simulink model "attempt_at_model_final"  (R2024a)
settings: Solver=FixedStepDiscrete  StartTime=0.0  StopTime=inf  FixedStep=0.01  RelTol=1e-3
model workspace (MAT data in the model file):
  SL_ROS_VariableLengthArrays_MaxSizes.CommonInfo.ArrayTruncateAction = 'EmitWarning'
  SL_ROS_VariableLengthArrays_MaxSizes.MsgTypeMap = containers.Map
  SL_ROS_VariableLengthArrays_MaxSizes.MsgTypeMap.serialization.keys = {'sensor_msgs/CompressedImage'}
  SL_ROS_VariableLengthArrays_MaxSizes.MsgTypeMap.serialization.values{1}(1).PropertyName = 'data'
  SL_ROS_VariableLengthArrays_MaxSizes.MsgTypeMap.serialization.values{1}(1).DataType = 'uint8'
  SL_ROS_VariableLengthArrays_MaxSizes.MsgTypeMap.serialization.values{1}(1).MaxLength = 87917
  SL_ROS_VariableLengthArrays_MaxSizes.MsgTypeMap.serialization.values{1}(2).PropertyName = 'format'
  SL_ROS_VariableLengthArrays_MaxSizes.MsgTypeMap.serialization.values{1}(2).DataType = 'uint8'
  SL_ROS_VariableLengthArrays_MaxSizes.MsgTypeMap.serialization.values{1}(2).MaxLength = 128
  SL_ROS_VariableLengthArrays_MaxSizes.MsgTypeMap.serialization.uniformity = 0
  SL_ROS_VariableLengthArrays_MaxSizes.MsgTypeMap.serialization.keyType = 'char'
  SL_ROS_VariableLengthArrays_MaxSizes.MsgTypeMap.serialization.valueType = 'any'
undefined symbols (not defined in the file): angular, linear
libraries: ros2lib x13, simulink x3, instrumentlib x1, etargetslib x1, vrlib x1, dspnetwork x1
settings Model: Creator=RedBlueBerry177  LastModifiedBy=ethan
settings OptimizationCC: EnhancedBackFolding=on  PassReuseOutputArgsAs=Individual arguments  ZeroExternalMemoryAtStartup=off  ZeroInternalMemoryAtStartup=off  MaxStackSize=64  OptimizeBlockOrder=speed  DifferentSizesBufferReuse=on  OptimizationCustomize=off  EfficientTunableParamExpr=on
settings DebuggingCC: ParameterTunabilityLossMsg=error
settings SFSimCC: MATLABDynamicMemAlloc=off  SimTargetLang=C++
settings RTWCC: Description=Embedded Coder  SystemTargetFile=ert.tlc  HardwareBoard=Robot Operating System 2 (ROS 2)  TLCOptions="-aInlineSetEventsForThisBaseRateFcn=TLC_FALSE -aSuppressMultiTaskScheduler=TLC_FALSE  -aRateBasedStepFcn=0"  TemplateMakefile=ert_default_tmf  Toolchain=Colcon Tools  TargetLang=C++  GPUComputeCapability=3.5
settings CodeAppCC: ForceParamTrailComments=on  IgnoreCustomStorageClasses=off  OperatorAnnotations=on  SimulinkDataObjDesc=on  SFDataObjDesc=on  InsertBlockDesc=on
settings ERTTargetCC: CodeInterfacePackaging=C++ class  RootIOFormat=Structure reference

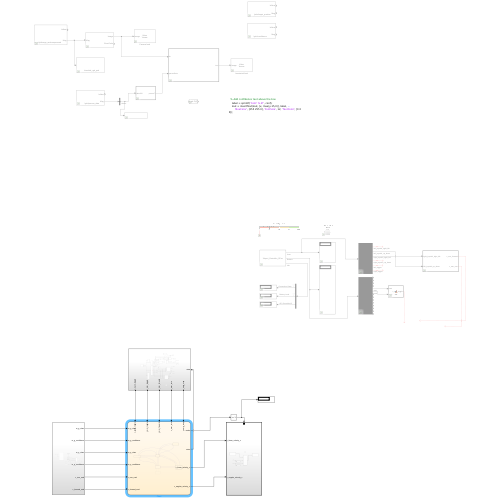
[thumbnail: Simulink's stored preview of the top-level diagram]
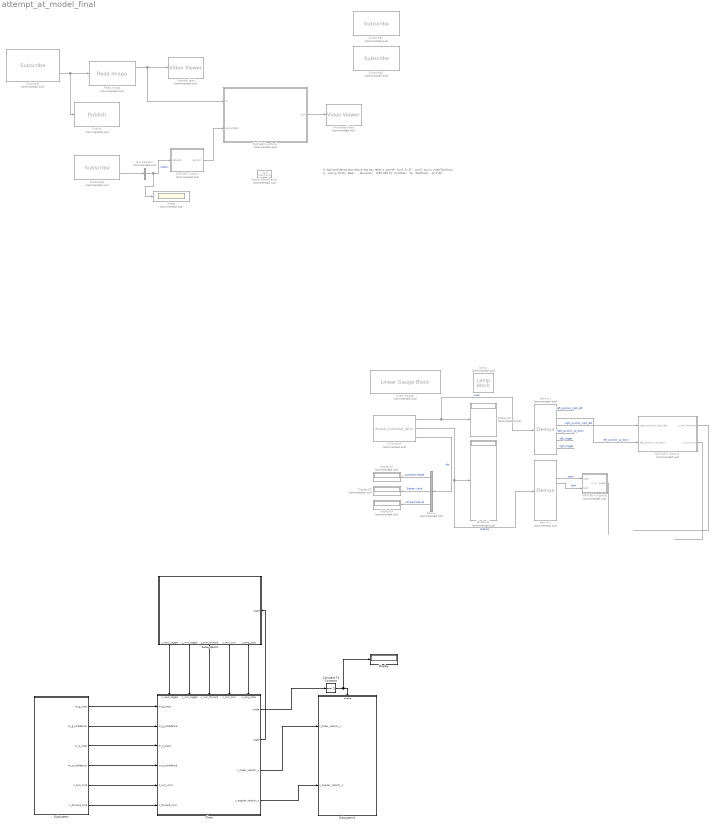
== system attempt_at_model_final ==
  note: % Add confidence text above the box
      | label = sprintf( 'Conf: %.2f' , conf);
      | Iout = insertText(Iout, [x, max(y-15,0)], label, ...
      | 'BoxColor' , [255 255 0], 'FontSize' , 12, 'TextColor' , [0 0 0]);
  Annotated feed : VideoViewer  Commented=on  FigPos=[1005 760 624 399]
  Bus Selector : BusSelector  Commented=on  OutputSignals=data
  Camera feed : VideoViewer  Commented=on  FigPos=[409 769 608 539]
  Chart : Stateflow chart  TreatAsAtomicUnit=on
      settings: PortSchema="{\"entries\":[{\"content\":{\"sides\":[{\"content\":{\"connectorIds\":[\"In5\",\"In6\",\"In7\",\"In8\",\"In9\",\"In10\"]},\"type\":\"ConnectorPlacement.EquallySpacedRectSide\",\"uuid\":\"6869af31-0483-4a0d-a5aa-348304382b03\"},{\"content\":{\"connectorIds\":[\"Out3\",\"Out4\",\"Out1\",\"Out2\"],\"side\":\"RIGHT\"},\"type\":\"ConnectorPlacement.EquallySpacedRectSide\",\"uuid\":\"19448461-0885-46d3-901b-79cbd3d2f2eb\"},{\"content\":{\"connectorIds\":[\"In11\",\"In3\",\"In1\",\"In2\",\"In4\"],\"side\":\"TOP\"},\"type\":\"ConnectorPlacement.EquallySpacedRectSide\",\"uuid\":\"dcdfc426-3300-4bb7-b0c9-b15241839ab0\"}]},\"type\":\"ConnectorPlacement.EquallySpacedConnector\",\"uuid\":\"e0f68e20-794f-48c9-96e4-1765267eb054\"}],\"packageUris\":[\"http://schema.mathworks.com/mf0/Connector/R2020b\"],\"version\":\"1.0\"}"
  Compare To Constant : simulink/Logic and Bit Operations/Compare To Constant  relop===  const=1  OutDataTypeStr=boolean
  Demux : Demux  Commented=on  Outputs=3
  Demux1 : Demux  Commented=on  Outputs=6
  Demux2 : Demux  Commented=on  Outputs=14
  Display : Display
  Display{30..34} (5 alike) : Display  Commented=on
  Lamp : LampBlock  Commented=on
  Linear Gauge : LinearGaugeBlock  Commented=on  TickInterval=25
  MATLAB Function : MATLAB Function  Commented=on  TreatAsAtomicUnit=on
  MATLAB Function1 : MATLAB Function  Commented=on  TreatAsAtomicUnit=on
  MATLAB Function5 : MATLAB Function  Commented=on  TreatAsAtomicUnit=on
  MATLAB Function6 : MATLAB Function  Commented=on  TreatAsAtomicUnit=on
  Publish : ros2lib/Publish  Commented=on  topicSource=Specify your own  topic=/simulink_rgb_pub  messageType=sensor_msgs/CompressedImage  QOSHistory=Keep last  QOSDepth=1  QOSReliability=Reliable  QOSDurability=Volatile  QOSDeadline=Inf  QOSLifespan=Inf  QOSLiveliness=Automatic  QOSLeaseDuration=Inf  QOSAvoidROSNamespaceConventions=off
  Read Image : ros2lib/Read Image  Commented=on  MaximumImageSize=[480,640]  ImageEncoding=rgb8  ShowAlphaOutput=off  ShowErrorCodeOutput=on  VariableSizeOutputs=off
  S-Function : S-Function  Commented=on  FunctionName=XInput_Controller_SFun  Parameters=1  SFunctionDeploymentMode=off  EnableBusSupport=off
  Scope : Scope  Commented=on
  Signal Specification : SignalSpecification  Commented=on  OutDataTypeStr=single  Dimensions=[1 7]
  Subscribe : ros2lib/Subscribe  Commented=on  topicSource=Select from ROS network  topic=/depth_cam/rgb/image_raw/compressed  messageType=sensor_msgs/CompressedImage  sampleTime=-1  QOSHistory=Keep last  QOSDepth=1  QOSReliability=Best effort  QOSDurability=Volatile  QOSDeadline=Inf  QOSLifespan=Inf  QOSLiveliness=Automatic  QOSLeaseDuration=Inf  QOSAvoidROSNamespaceConventions=off
  Subscribe1 : ros2lib/Subscribe  Commented=on  topicSource=Select from ROS network  topic=/yolo/target_position  messageType=geometry_msgs/Point  sampleTime=-1  QOSHistory=Keep last  QOSDepth=1  QOSReliability=Reliable  QOSDurability=Volatile  QOSDeadline=Inf  QOSLifespan=Inf  QOSLiveliness=Automatic  QOSLeaseDuration=Inf  QOSAvoidROSNamespaceConventions=off
  Subscribe2 : ros2lib/Subscribe  Commented=on  topicSource=Select from ROS network  topic=/yolo/confidence  messageType=std_msgs/Float32  sampleTime=-1  QOSHistory=Keep last  QOSDepth=1  QOSReliability=Reliable  QOSDurability=Volatile  QOSDeadline=Inf  QOSLifespan=Inf  QOSLiveliness=Automatic  QOSLeaseDuration=Inf  QOSAvoidROSNamespaceConventions=off
  Subscribe3 : ros2lib/Subscribe  Commented=on  topicSource=Select from ROS network  topic=/yolo/person_data  messageType=std_msgs/Float32MultiArray  sampleTime=-1  QOSHistory=Keep last  QOSDepth=1  QOSReliability=Reliable  QOSDurability=Volatile  QOSDeadline=Inf  QOSLifespan=Inf  QOSLiveliness=Automatic  QOSLeaseDuration=Inf  QOSAvoidROSNamespaceConventions=off
  Subsystem : Subsystem
  Subsystem1 : Subsystem
  Subsystem2 : Subsystem
      settings: PortSchema="{\"entries\":[{\"content\":{\"sides\":[{\"content\":{},\"type\":\"ConnectorPlacement.EquallySpacedRectSide\",\"uuid\":\"85a25dc4-4ac2-493d-892d-263cb269b942\"},{\"content\":{\"connectorIds\":[\"In1\"],\"side\":\"RIGHT\"},\"type\":\"ConnectorPlacement.EquallySpacedRectSide\",\"uuid\":\"9ba6428f-e6fb-4336-a01e-053275131db5\"},{\"content\":{\"side\":\"TOP\"},\"type\":\"ConnectorPlacement.EquallySpacedRectSide\",\"uuid\":\"19c386df-5b9f-4043-add8-e382a7c76f3c\"},{\"content\":{\"connectorIds\":[\"Out1\",\"Out2\",\"Out3\",\"Out4\",\"Out5\"],\"side\":\"BOTTOM\"},\"type\":\"ConnectorPlacement.EquallySpacedRectSide\",\"uuid\":\"ad9dad01-2690-4610-af5e-2189b0573909\"}]},\"type\":\"ConnectorPlacement.EquallySpacedConnector\",\"uuid\":\"50284396-e3f7-42bc-a456-730720622e26\"}],\"packageUris\":[\"http://schema.mathworks.com/mf0/Connector/R2020b\"],\"version\":\"1.0\"}"
  wires:
  Subscribe/2 -> Publish/1, Read Image/1
  Read Image/1 -> MATLAB Function1/1(Iin), Camera feed/1
  MATLAB Function1/1(Iout) -> Annotated feed/1
  Subscribe3/2 -> Bus Selector/1
  Bus Selector/1 -> Scope/1, MATLAB Function/1(data128)  "<data>"
  MATLAB Function/1(person7) -> MATLAB Function1/2(personData)
  Subsystem/1(m_g_class) -> Chart/5(m_g_class)
  Subsystem/2(m_g_confidence) -> Chart/6(m_g_confidence)
  Subsystem/3(m_p_class) -> Chart/7(m_p_class)
  Subsystem/4(m_p_confidence) -> Chart/8(m_p_confidence)
  Chart/1(c_linear_velocity_x) -> Subsystem1/1(c_linear_velocity_x)
  Subsystem/5(c_turn_cmd) -> Chart/9(c_turn_cmd)
  Subsystem/6(c_forward_cmd) -> Chart/10(c_forward_cmd)
  Chart/2(c_angular_velocity_z) -> Subsystem1/2(c_angular_velocity_z)
  MATLAB Function5/1(c_mm_forward) -> ?
  MATLAB Function5/2(c_mm_turn) -> ?
  MATLAB Function6/1(c_mm_toggle) -> ?
  Demux/2 -> Display33/1  "Battery Level"
  S-Function/2 -> Demux2/1, Display31/1  "Buttons"
  S-Function/1 -> Demux1/1, Display30/1  "Axes"
  S-Function/3 -> Demux/1  "Info"
  Demux/1 -> Display32/1  "Connection State"
  Demux/3 -> Display34/1  "API Controller ID"
  Demux1/2 -> MATLAB Function5/2(left_joystick_up_down)  "left_joystick_up_down"
  Demux1/3 -> MATLAB Function5/1(right_joystick_right_left)  "right_joystick_right_left"
  Demux1/4 -> ?  "right_joystick_up_down"
  Demux1/5 -> ?  "left_trigger"
  Demux1/6 -> ?  "right_trigger"
  Demux2/5 -> MATLAB Function6/1(start)  "start"
  Demux2/6 -> MATLAB Function6/2(back)  "back"
  Demux1/1 -> ?  "left_joystick_right_left"
  Subsystem2/2(c_mm_toggle) -> Chart/3(c_mm_toggle)
  Subsystem2/3(c_mm_forward) -> Chart/1(c_mm_forward)
  Subsystem2/4(c_mm_turn) -> Chart/2(c_mm_turn)
  Subsystem2/5(c_emg_stop) -> Chart/4(c_emg_stop)
  Subsystem2/1(c_nav2_toggle) -> Chart/11(c_nav2_toggle)
  Chart/3(mode) -> Compare To Constant/1
  Compare To Constant/1 -> Display/1, Subsystem1/Enable
  Chart/4(state) -> Subsystem2/1(state)

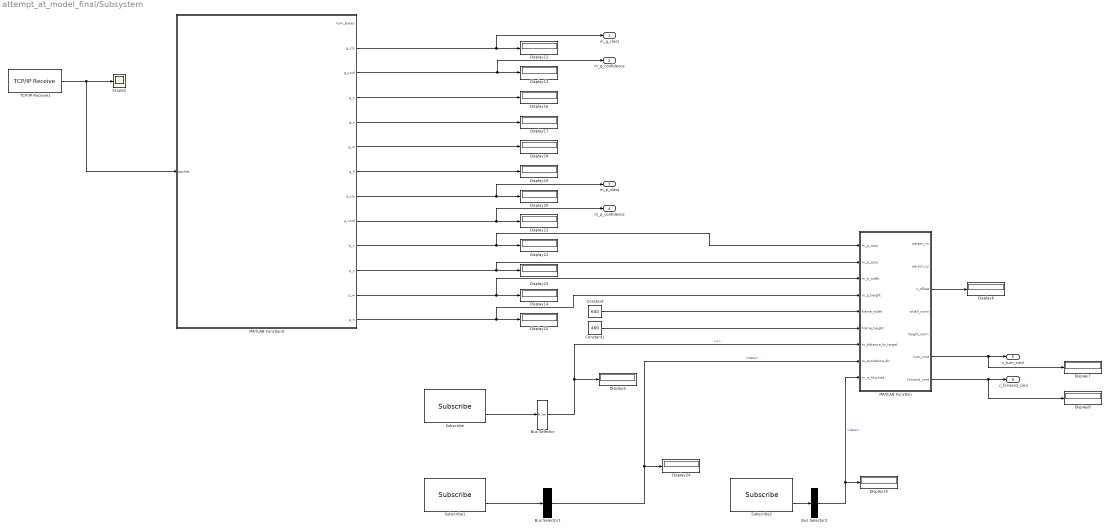
== system attempt_at_model_final/Subsystem ==
  Bus Selector : BusSelector  OutputSignals=pose.position.x
  Bus Selector1 : BusSelector  OutputSignals=data
  Bus Selector2 : BusSelector  OutputSignals=data
  Constant : Constant  Value=640
  Constant1 : Constant  Value=480
  Display{6..9,12..25} (18 alike) : Display
  MATLAB Function : MATLAB Function  TreatAsAtomicUnit=on
  MATLAB Function3 : MATLAB Function  TreatAsAtomicUnit=on
  Scope2 : Scope
  Subscribe : ros2lib/Subscribe  topicSource=Select from ROS network  topic=/person_pose  messageType=geometry_msgs/PoseStamped  sampleTime=-1  QOSHistory=Keep last  QOSDepth=1  QOSReliability=Reliable  QOSDurability=Volatile  QOSDeadline=Inf  QOSLifespan=Inf  QOSLiveliness=Automatic  QOSLeaseDuration=Inf  QOSAvoidROSNamespaceConventions=off
  Subscribe1 : ros2lib/Subscribe  topicSource=Select from ROS network  topic=/avoidance_dir  messageType=std_msgs/Int32  sampleTime=-1  QOSHistory=Keep last  QOSDepth=1  QOSReliability=Reliable  QOSDurability=Volatile  QOSDeadline=Inf  QOSLifespan=Inf  QOSLiveliness=Automatic  QOSLeaseDuration=Inf  QOSAvoidROSNamespaceConventions=off
  Subscribe2 : ros2lib/Subscribe  topicSource=Select from ROS network  topic=/is_blocked  messageType=std_msgs/Bool  sampleTime=-1  QOSHistory=Keep last  QOSDepth=1  QOSReliability=Reliable  QOSDurability=Volatile  QOSDeadline=Inf  QOSLifespan=Inf  QOSLiveliness=Automatic  QOSLeaseDuration=Inf  QOSAvoidROSNamespaceConventions=off
  TCP/IP Receive1 : instrumentlib/TCP//IP Receive  Host=127.0.0.1  Port=5005  DataSize=[52, 1]  DataType=uint8  ASCIIFormatting=%f  Terminator=LF  CustomTerminator=10  ByteOrder=big-endian  EnableBlockingMode=on  Timeout=1000  SampleTime=0.01  SimulateUsing=Interpreted execution
  m_g_class : Outport
  m_g_confidence : Outport  Port=2
  m_p_class : Outport  Port=3
  m_p_confidence : Outport  Port=4
  c_turn_cmd : Outport  Port=5
  c_forward_cmd : Outport  Port=6
  wires:
  MATLAB Function3/9(p_conf) -> m_p_confidence/1, Display21/1
  MATLAB Function3/6(g_w) -> Display18/1
  MATLAB Function3/4(g_x) -> Display16/1
  MATLAB Function3/13(p_h) -> MATLAB Function/4(m_p_height), Display15/1
  MATLAB Function3/10(p_x) -> MATLAB Function/1(m_p_xpos), Display22/1
  MATLAB Function3/7(g_h) -> Display19/1
  MATLAB Function3/8(p_cls) -> m_p_class/1, Display20/1
  MATLAB Function3/11(p_y) -> MATLAB Function/2(m_p_ypos), Display23/1
  MATLAB Function3/3(g_conf) -> m_g_confidence/1, Display13/1
  MATLAB Function3/2(g_cls) -> m_g_class/1, Display12/1
  MATLAB Function3/5(g_y) -> Display17/1
  TCP/IP Receive1/1 -> MATLAB Function3/1(packet), Scope2/1
  MATLAB Function3/12(p_w) -> MATLAB Function/3(m_p_width), Display14/1
  Constant/1 -> MATLAB Function/5(frame_width)
  Constant1/1 -> MATLAB Function/6(frame_height)
  MATLAB Function/3(x_offset) -> Display6/1
  MATLAB Function/6(turn_cmd) -> Display7/1, c_turn_cmd/1
  MATLAB Function/7(forward_cmd) -> Display8/1, c_forward_cmd/1
  Subscribe/2 -> Bus Selector/1
  Bus Selector/1 -> MATLAB Function/7(m_distance_to_target), Display9/1  "<x>"
  Subscribe1/2 -> Bus Selector1/1
  Subscribe2/2 -> Bus Selector2/1
  Bus Selector1/1 -> Display24/1, MATLAB Function/8(m_avoidance_dir)  "<data>"
  Bus Selector2/1 -> MATLAB Function/9(m_is_blocked), Display25/1  "<data>"

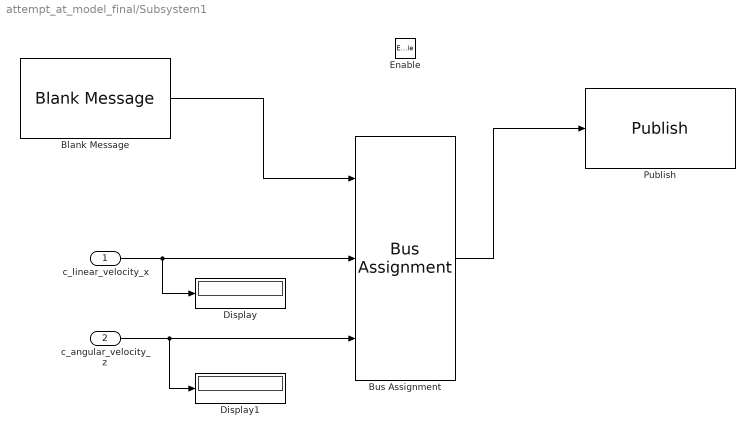
== system attempt_at_model_final/Subsystem1 ==
  c_linear_velocity_x : Inport
  c_angular_velocity_z : Inport  Port=2
  Enable : EnablePort
  Blank Message : ros2lib/Blank Message  messageClass=Message  entityType=geometry_msgs/Twist  messageType=geometry_msgs/Twist  SampleTime=inf
  Bus Assignment : BusAssignment  AssignedSignals=linear.x,angular.z
  Display : Display
  Display1 : Display
  Publish : ros2lib/Publish  topicSource=Select from ROS network  topic=/controller/cmd_vel  messageType=geometry_msgs/Twist  QOSHistory=Keep last  QOSDepth=1  QOSReliability=Reliable  QOSDurability=Volatile  QOSDeadline=Inf  QOSLifespan=Inf  QOSLiveliness=Automatic  QOSLeaseDuration=Inf  QOSAvoidROSNamespaceConventions=off
  wires:
  Blank Message/1 -> Bus Assignment/1
  c_linear_velocity_x/1 -> Display/1, Bus Assignment/2
  Bus Assignment/1 -> Publish/1
  c_angular_velocity_z/1 -> Display1/1, Bus Assignment/3

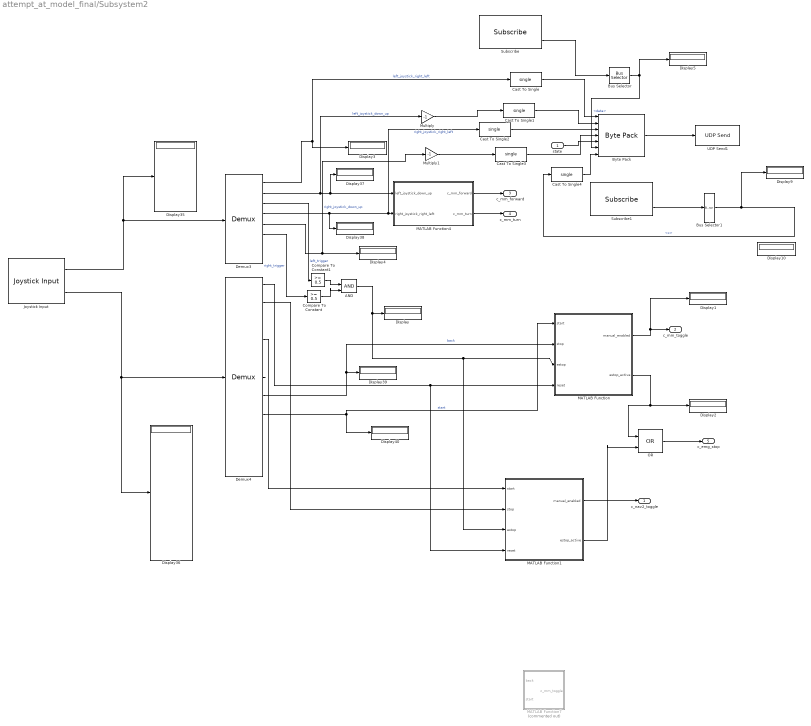
== system attempt_at_model_final/Subsystem2 ==
  state : Inport
  AND : Logic  IconShape=distinctive  AllPortsSameDT=off  OutDataTypeStr=boolean
  Bus Selector : BusSelector  OutputSignals=data
  Bus Selector1 : BusSelector  OutputSignals=pose.position.x
  Byte Pack : etargetslib/Byte Pack  datatypes={'single','single','single','single','uint8','uint16','single'}  byteAlign=1
  Cast To Single{,1..4} (5 alike) : DataTypeConversion  OutDataTypeStr=single  SaturateOnIntegerOverflow=off  RndMeth=Floor
  Compare To Constant : simulink/Logic and Bit Operations/Compare To Constant  relop=>=  const=0.5  OutDataTypeStr=boolean
  Compare To Constant1 : simulink/Logic and Bit Operations/Compare To Constant  relop=>=  const=0.5  OutDataTypeStr=boolean
  Demux3 : Demux  Outputs=8
  Demux4 : Demux  Outputs=11
  Display{,1..5,9..10,35..40} (14 alike) : Display
  Joystick Input : vrlib/Joystick Input  joyid=1  adjustports=on  forcefeed=off
  MATLAB Function : MATLAB Function  TreatAsAtomicUnit=on
  MATLAB Function1 : MATLAB Function  TreatAsAtomicUnit=on
  MATLAB Function4 : MATLAB Function  TreatAsAtomicUnit=on
  MATLAB Function7 : MATLAB Function  Commented=on  TreatAsAtomicUnit=on
  Multiply : Gain  Gain=-1
  Multiply1 : Gain  Gain=-1
  OR : Logic  Operator=OR  IconShape=distinctive  AllPortsSameDT=off  OutDataTypeStr=boolean
  Subscribe : ros2lib/Subscribe  topicSource=Select from ROS network  topic=/ros_robot_controller/battery  messageType=std_msgs/UInt16  sampleTime=-1  QOSHistory=Keep last  QOSDepth=1  QOSReliability=Reliable  QOSDurability=Volatile  QOSDeadline=Inf  QOSLifespan=Inf  QOSLiveliness=Automatic  QOSLeaseDuration=Inf  QOSAvoidROSNamespaceConventions=off
  Subscribe1 : ros2lib/Subscribe  topicSource=Select from ROS network  topic=/person_pose  messageType=geometry_msgs/PoseStamped  sampleTime=-1  QOSHistory=Keep last  QOSDepth=1  QOSReliability=Reliable  QOSDurability=Volatile  QOSDeadline=Inf  QOSLifespan=Inf  QOSLiveliness=Automatic  QOSLeaseDuration=Inf  QOSAvoidROSNamespaceConventions=off
  UDP Send1 : dspnetwork/UDP Send  remoteURL='127.0.0.1'  remotePort=5011  localURL='0.0.0.0'  localPortSource=Automatically determine  localPort=-1  sendBufferSize=23  sampletime=-1  blockPlatform=[]  separateLengthPort=0
      settings: LibrarySourceBlock=dspsnks4/UDP Send
  c_nav2_toggle : Outport
  c_mm_toggle : Outport  Port=2
  c_mm_forward : Outport  Port=3
  c_mm_turn : Outport  Port=4
  c_emg_stop : Outport  Port=5
  wires:
  Demux3/2 -> Multiply/1, MATLAB Function4/1(left_joystick_down_up), Display37/1  "left_joystick_down_up"
  Demux4/6 -> ?
  Joystick Input/2 -> Display36/1, Demux4/1
  Demux3/1 -> Cast To Single/1, Display3/1  "left_joystick_right_left"
  Joystick Input/1 -> Display35/1, Demux3/1
  MATLAB Function4/2(c_mm_turn) -> c_mm_turn/1
  Demux3/3 -> Compare To Constant1/1  "left_trigger"
  MATLAB Function4/1(c_mm_forward) -> c_mm_forward/1
  Demux3/4 -> Display38/1, Cast To Single2/1, MATLAB Function4/2(right_joystick_right_left)  "right_joystick_right_left"
  Demux3/6 -> Compare To Constant/1  "right_trigger"
  Demux3/5 -> Multiply1/1, Display4/1  "right_joystick_down_up"
  Demux4/4 -> MATLAB Function1/1(start)
  Demux4/8 -> Display40/1, MATLAB Function/1(start)  "start"
  Demux4/7 -> MATLAB Function/2(stop), Display39/1  "back"
  AND/1 -> MATLAB Function1/3(estop), MATLAB Function/3(estop), Display/1
  Compare To Constant1/1 -> AND/1
  Compare To Constant/1 -> AND/2
  MATLAB Function/1(manual_enabled) -> Display1/1, c_mm_toggle/1
  MATLAB Function/2(estop_active) -> Display2/1, OR/1
  Demux4/1 -> MATLAB Function1/4(reset), MATLAB Function/4(reset)
  MATLAB Function1/1(manual_enabled) -> c_nav2_toggle/1
  Demux4/2 -> MATLAB Function1/2(stop)
  MATLAB Function1/2(estop_active) -> OR/2
  OR/1 -> c_emg_stop/1
  Multiply/1 -> Cast To Single1/1
  Multiply1/1 -> Cast To Single3/1
  state/1 -> Byte Pack/5
  Byte Pack/1 -> UDP Send1/1
  Cast To Single/1 -> Byte Pack/1
  Cast To Single1/1 -> Byte Pack/2
  Cast To Single2/1 -> Byte Pack/3
  Cast To Single3/1 -> Byte Pack/4
  Subscribe/2 -> Bus Selector/1
  Bus Selector/1 -> Byte Pack/6, Display5/1  "<data>"
  Bus Selector1/1 -> Cast To Single4/1, Display9/1  "<x>"
  Subscribe1/2 -> Bus Selector1/1
  Cast To Single4/1 -> Byte Pack/7

== matlab function attempt_at_model_final/MATLAB Function ==
  data: data128 input; person7 output
function person7 = slicePersonData(data128)
% data128: [128x1] or [1x128]
person7 = reshape(data128(1:7), 1, 7);
end

== matlab function attempt_at_model_final/Subsystem2/MATLAB Function4 ==
  data: left_joystick_down_up input; c_mm_forward output; c_mm_turn output; right_joystick_right_left input
function [c_mm_forward, c_mm_turn] = fcn(left_joystick_down_up, right_joystick_right_left)
%#codegen


deadzone = 0.2;


max_lin_vel = 0.25;
max_ang_vel = 0.3;

x = right_joystick_right_left;
y = left_joystick_down_up;

if(abs(x) < deadzone)
    x = 0;
end

if(abs(y) < deadzone)
    y = 0;
end

c_mm_forward = -y * max_lin_vel;
c_mm_turn = -x * max_ang_vel;



end

== stateflow chart attempt_at_model_final/Chart ==
  state Path_Planning_and_Navigation
    state = 4
  state Initial
    mode = 1
  state Manual_Mode
    c_linear_velocity_x = c_mm_forward;
    c_angular_velocity_z = c_mm_turn;
    state = 3
  state Follow
    c_linear_velocity_x = c_forward_cmd;
    c_angular_velocity_z = c_turn_cmd;
    state = 2
  state Idle
    c_linear_velocity_x = 0.0;
    c_angular_velocity_z = 0.0;
    state = 1
  state Mapping_and_Localization [commented out]
  Path_Planning_and_Navigation -> Initial [order 2] : [c_emg_stop == 1]
      | {c_linear_velocity_x = 0,
      | c_angular_velocity_z = 0,
      | mode = 1, state = 5}
  Path_Planning_and_Navigation -> Initial [order 1] : [(c_nav2_toggle == 0) & (c_emg_stop == 0)]
      | {mode = 1, state = 0}
  Initial -> Path_Planning_and_Navigation [order 2] : [c_nav2_toggle == 1]{mode = 2}
  Follow -> Manual_Mode [order 2] : [c_mm_toggle ==1]
  Manual_Mode -> Initial [order 2] : [c_emg_stop == 1]{c_linear_velocity_x = 0, c_angular_velocity_z = 0, state = 5}
  (default) -> Initial : {state = 0}
  Follow -> Initial [order 3] : [c_emg_stop == 1]
      | {c_linear_velocity_x = 0,
      | c_angular_velocity_z = 0,
      | state = 5}
  Initial -> Manual_Mode [order 1] : [c_mm_toggle == 1]
  Manual_Mode -> Initial [order 3] : [(c_mm_toggle == 0) & (m_p_class == 0)]{state = 0}
  Follow -> Initial [order 4] : [m_p_class == 0]{state = 0}
  Idle -> Initial [order 3] : [c_emg_stop == 1]
      | {c_linear_velocity_x = 0,
      | c_angular_velocity_z = 0,
      | state = 5}
  Initial -> Idle [order 3] : [(m_g_class == 9) & (m_p_class ==1) & (c_emg_stop == 0)]
  Manual_Mode -> Idle [order 1] : [(c_mm_toggle == 0) & (m_p_class == 1) & (c_emg_stop == 0)]
  Idle -> Manual_Mode [order 2] : [c_mm_toggle == 1]
  Idle -> Follow [order 1] : [m_g_class == 20]
  Follow -> Idle [order 1] : [(m_g_class == 13)]
  Idle -> Mapping_and_Localization [commented out] : [m_g_class == 13]
  Mapping_and_Localization -> Idle [commented out]
  data: c_mm_forward input; c_mm_turn input; c_mm_toggle input; c_emg_stop input; m_g_class input; m_g_confidence input; m_p_class input; m_p_confidence input; c_linear_velocity_x output; c_turn_cmd input; c_forward_cmd input; c_angular_velocity_z output; c_nav2_toggle input; mode output; state output

== matlab function attempt_at_model_final/Subsystem2/MATLAB Function7 ==
  data: back input; c_mm_toggle output; start input
function c_mm_toggle = fcn(back, start)
%#codegen
% Manual control enable latch
% start = 1 → enable manual mode
% back  = 1 → disable manual mode

persistent manual_enabled

% Initialize once
if isempty(manual_enabled)
    manual_enabled = false;
end

% Update logic
if start
    manual_enabled = true;
elseif back
    manual_enabled = false;
end

% Output
c_mm_toggle = manual_enabled;

end

== matlab function attempt_at_model_final/Subsystem/MATLAB Function3 ==
  data: num_boxes output uint32 size=1; packet input; g_cls output int32 size=1; g_conf output single size=1; g_x output single size=1; g_y output single size=1; g_w output single size=1; g_h output single size=1; p_cls output int32 size=1; p_conf output single size=1; p_x output single size=1; p_y output single size=1; p_w output single size=1; p_h output single size=1
function [num_boxes, g_cls, g_conf, g_x, g_y, g_w, g_h, p_cls, p_conf, p_x, p_y, p_w, p_h] = parse_packet(packet)

num_boxes = typecast(packet(1:4), 'uint32');

% Person box
p_cls  = typecast(packet(5:8), 'int32');
p_conf = typecast(packet(9:12), 'single');
p_x    = typecast(packet(13:16), 'single');
p_y    = typecast(packet(17:20), 'single');
p_w    = typecast(packet(21:24), 'single');
p_h    = typecast(packet(25:28), 'single');

% Gesture box
g_cls  = typecast(packet(29:32), 'int32');
g_conf = typecast(packet(33:36), 'single');
g_x    = typecast(packet(37:40), 'single');
g_y    = typecast(packet(41:44), 'single');
g_w    = typecast(packet(45:48), 'single');
g_h    = typecast(packet(49:52), 'single');
end

== matlab function attempt_at_model_final/Subsystem/MATLAB Function ==
  data: m_p_xpos input; person_cx output; m_p_ypos input; m_p_width input; m_p_height input; frame_width input; frame_height input; person_cy output; x_offset output; width_norm output; height_norm output; turn_cmd output; forward_cmd output; m_distance_to_target input; m_avoidance_dir input; m_is_blocked input
function [person_cx, person_cy, x_offset, width_norm, height_norm, turn_cmd, forward_cmd] = compute_person_controls(m_p_xpos, m_p_ypos, m_p_width, m_p_height, frame_width, frame_height, m_distance_to_target, m_avoidance_dir, m_is_blocked)

% Initialize outputs to zero to prevent 'drifting'
turn_cmd = 0.0;
forward_cmd = 0.0;

% Compute standard YOLO values
person_cx = m_p_xpos + m_p_width/2;
person_cy = m_p_ypos + m_p_height/2;
x_offset = person_cx - frame_width/2;
width_norm = m_p_width / frame_width;
height_norm = m_p_height / frame_height;

% ------------------------
% OBSTACLE AVOIDANCE (Priority 1)
% ------------------------
if m_is_blocked > 0.5
    forward_cmd = -0.1;
    if m_avoidance_dir == 1
        turn_cmd = -0.4;  
    elseif m_avoidance_dir == 2
        turn_cmd = 0.4; 
    else
        turn_cmd = 0.4; 
    end

% ------------------------
% NORMAL PERSON FOLLOWING (Priority 2)
% ------------------------
else
    % Turning logic
    x_threshold = 40; 
    if x_offset < -x_threshold
        turn_cmd = 0.25; 
    elseif x_offset > x_threshold
        turn_cmd = -0.25; 
    else
        turn_cmd = 0.0;
    end

    % Forward logic
    if m_distance_to_target > 1
        forward_cmd = 0.18;   
    elseif m_distance_to_target < 0.6
        forward_cmd = 0.0;      
    else
        forward_cmd = 0.0;      
    end

    if width_norm > 0.85
        forward_cmd = 0.0;
    end
end

turn_cmd = double(turn_cmd);
forward_cmd = double(forward_cmd);

end

== matlab function attempt_at_model_final/Subsystem2/MATLAB Function ==
  data: start input; manual_enabled output; stop input; estop input; estop_active output; reset input
function [manual_enabled, estop_active] = fcn(start, stop, estop, reset)
%#codegen

persistent prev_start prev_stop prev_estop prev_reset
persistent manual_state estop_state

if isempty(manual_state)
    manual_state = false;
    estop_state  = false;
    prev_start = false;
    prev_stop  = false;
    prev_estop = false;
    prev_reset = false;
end

% Convert to logical
start = (start == 1);
stop  = (stop  == 1);
estop = (estop == 1);
reset = (reset == 1);

% Edge detection
start_edge = start && ~prev_start;
stop_edge  = stop  && ~prev_stop;
estop_edge = estop && ~prev_estop;
reset_edge = reset && ~prev_reset;

% --- E-STOP ---
if estop_edge
    estop_state = true;
elseif reset_edge
    estop_state = false;
end

% --- MANUAL ---
if estop_state
    manual_state = false;
elseif start_edge
    manual_state = true;
elseif stop_edge
    manual_state = false;
end

% Save previous
prev_start = start;
prev_stop  = stop;
prev_estop = estop;
prev_reset = reset;

manual_enabled = manual_state;
estop_active   = estop_state;

end

== matlab function attempt_at_model_final/Subsystem2/MATLAB Function1 ==
  data: start input; manual_enabled output; stop input; estop input; estop_active output; reset input
function [manual_enabled, estop_active] = fcn(start, stop, estop, reset)
%#codegen

persistent prev_start prev_stop prev_estop prev_reset
persistent manual_state estop_state

if isempty(manual_state)
    manual_state = false;
    estop_state  = false;
    prev_start = false;
    prev_stop  = false;
    prev_estop = false;
    prev_reset = false;
end

% Convert to logical
start = (start == 1);
stop  = (stop  == 1);
estop = (estop == 1);
reset = (reset == 1);

% Edge detection
start_edge = start && ~prev_start;
stop_edge  = stop  && ~prev_stop;
estop_edge = estop && ~prev_estop;
reset_edge = reset && ~prev_reset;

% --- E-STOP ---
if estop_edge
    estop_state = true;
elseif reset_edge
    estop_state = false;
end

% --- MANUAL ---
if estop_state
    manual_state = false;
elseif start_edge
    manual_state = true;
elseif stop_edge
    manual_state = false;
end

% Save previous
prev_start = start;
prev_stop  = stop;
prev_estop = estop;
prev_reset = reset;

manual_enabled = manual_state;
estop_active   = estop_state;

end

== matlab function attempt_at_model_final/MATLAB Function5 ==
  data: c_mm_forward output; c_mm_turn output; right_joystick_right_left input; left_joystick_up_down input
function [c_mm_forward, c_mm_turn] = fcn(right_joystick_right_left, left_joystick_up_down)
%#codegen


deadzone = 0.2;


max_lin_vel = 0.2;
max_ang_vel = 0.3;

x = right_joystick_right_left;
y = left_joystick_up_down;

if(abs(x) < deadzone)
    x = 0;
end

if(abs(y) < deadzone)
    y = 0;
end

c_mm_forward = y * max_lin_vel;
c_mm_turn = -x * max_ang_vel;



end

== matlab function attempt_at_model_final/MATLAB Function6 ==
  data: c_mm_toggle output; start input; back input
function c_mm_toggle = fcn(start, back)
%#codegen
% Manual control enable latch
% start = 1 → enable manual mode
% back  = 1 → disable manual mode

persistent manual_enabled

% Initialize once
if isempty(manual_enabled)
    manual_enabled = false;
end

% Update logic
if start
    manual_enabled = true;
elseif back
    manual_enabled = false;
end

% Output
c_mm_toggle = manual_enabled;

end

== matlab function attempt_at_model_final/MATLAB Function1 ==
  data: Iin input; Iout output uint8 size=[480 640 3]; personData input single size=[1 7]
function Iout = drawPersonBox(Iin, personData)
% Iin         : Input RGB image (HxWx3)
% personData  : 1x7 Float32 array [x y w h cx cy confidence]

Iout = Iin;  % start with the original image

% Extract data
x = personData(1);
y = personData(2);
w = personData(3);
h = personData(4);
cx = personData(5);
cy = personData(6);
conf = personData(7);

% Only draw if confidence > 0
if conf > 0
    % Draw rectangle around detected person
    Iout = insertShape(Iout, 'Rectangle', [x, y, w, h], ...
        'Color', [0 255 0], 'LineWidth', 3);

  


end
